simulink subsystem "VehicleDetectorMetrics"  (R2024b)
settings: Solver=VariableStepAuto  StartTime=0.0  StopTime=10.0  RelTol=1e-3
settings Model: Creator=The MathWorks, Inc.  LastModifiedBy=The MathWorks, Inc.
settings SolverCC: MaxZcPerStep=1
settings DebuggingCC: UnconnectedInputMsg=warning  UnconnectedOutputMsg=warning  UnconnectedLineMsg=warning  SubsystemReferenceDiagnosticForUnitTest=warning
settings ModelReferenceCC: EnableRefExpFcnMdlSchedulingChecks=on
settings RTWCC: GPUComputeCapability=3.5  DLArmComputeVersion=19.05

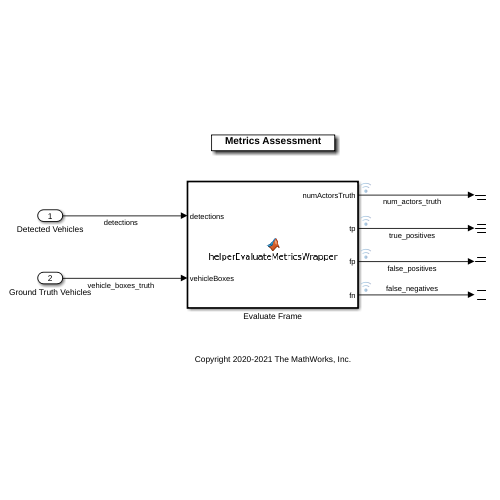
[thumbnail: Simulink's stored preview of the top-level diagram]
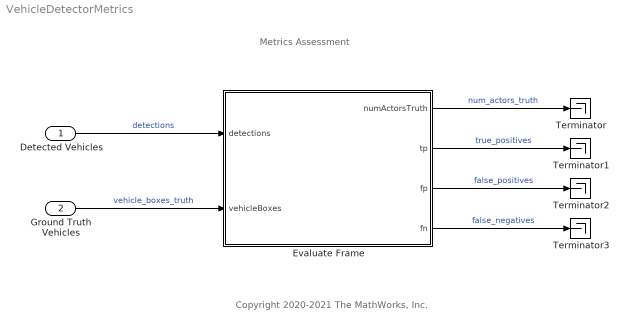
== system VehicleDetectorMetrics ==
  note: Metrics Assessment
  note: Copyright 2020-2021 The MathWorks, Inc.
  Detected Vehicles : Inport
  Ground Truth Vehicles : Inport  Port=2
  Evaluate Frame : MATLAB Function  TreatAsAtomicUnit=on
  Terminator{,1..3} (4 alike) : Terminator
  wires:
  Ground Truth Vehicles/1 -> Evaluate Frame/2(vehicleBoxes)  "vehicle_boxes_truth"
  Detected Vehicles/1 -> Evaluate Frame/1(detections)  "detections"
  Evaluate Frame/2(tp) -> Terminator1/1  "true_positives"
  Evaluate Frame/3(fp) -> Terminator2/1  "false_positives"
  Evaluate Frame/4(fn) -> Terminator3/1  "false_negatives"
  Evaluate Frame/1(numActorsTruth) -> Terminator/1  "num_actors_truth"

== matlab function VehicleDetectorMetrics/Evaluate Frame ==
  data: numActorsTruth output; tp output; fp output; fn output; detections input; vehicleBoxes input size=[20,4]
function [numActorsTruth, tp, fp, fn] ...
    = helperEvaluateMetricsWrapper(detections, vehicleBoxes)
% Wrapper function to call the helperEvaluateMetrics.

tp = 0;
fp = 0;
fn = 0;

% Output number of actors in truth for assessing metrics
numActorsTruth = size(vehicleBoxes(any(vehicleBoxes, 2), :),1);

coder.extrinsic('helperEvaluateMetrics');
 
[tp, fp, fn] = ...
    helperEvaluateMetrics(detections, vehicleBoxes);

end
